simulink model "GEMV_Stream_Ex2"  (R2025a)
settings: Solver=VariableStepAuto  StartTime=0.0  StopTime=100  RelTol=1e-3
undefined symbols (not defined in the file): Column, DUT, GEMV_Ex1_Stream, L, major, vsva1596, xcvc1702
libraries: aieUtilities x2, aieDSP x1, vmcUtilities x1
settings Model: Creator=sdegala  LastModifiedBy=sdegala
settings ModelReferenceCC: EnableRefExpFcnMdlSchedulingChecks=on
settings RTWCC: GPUComputeCapability=3.5

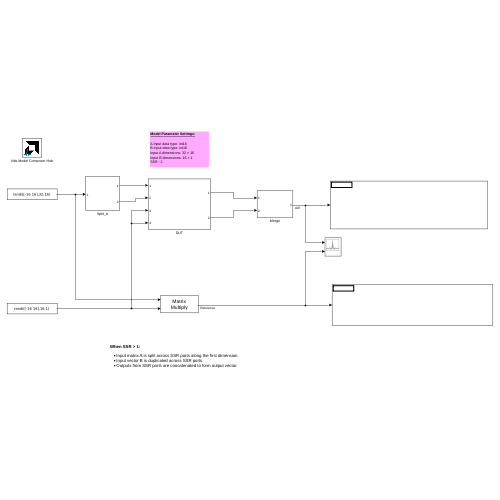
[thumbnail: Simulink's stored preview of the top-level diagram]
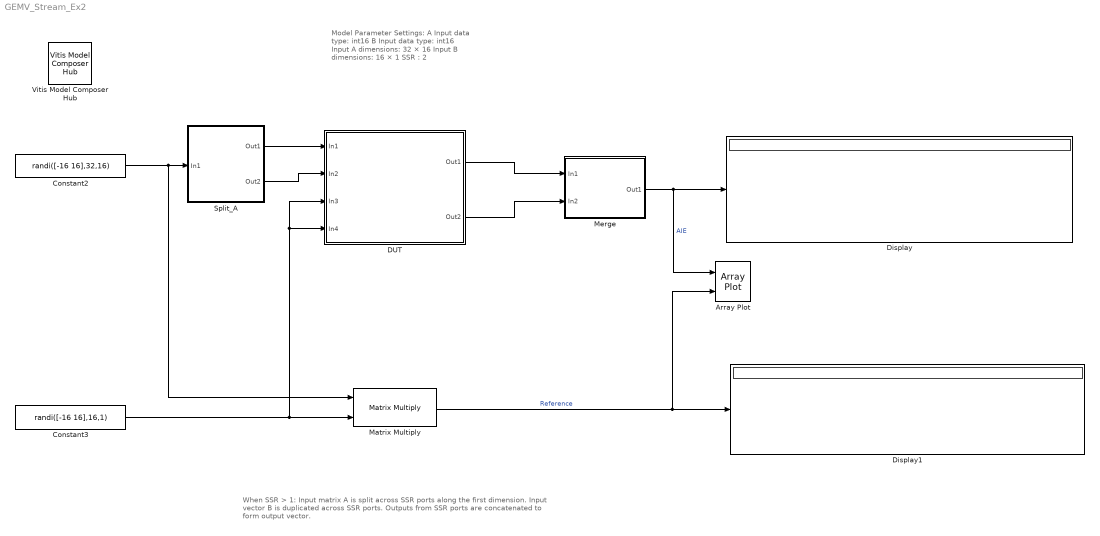
== system GEMV_Stream_Ex2 ==
  note: Model Parameter Settings:
      |
      | A Input data type: int16
      | B Input data type: int16
      | Input A dimensions: 32 × 16
      | Input B dimensions: 16 × 1
      | SSR : 2
  note: When SSR > 1:
      | Input matrix A is split across SSR ports along the first dimension.
      | Input vector B is duplicated across SSR ports.
      | Outputs from SSR ports are concatenated to form output vector.
  Array Plot : ArrayPlot  NumInputPorts=2  WindowPosition=[560.000000,350.000000,800.000000,500.000000,]  Visible=on  ScopeFrameLocation=window  YLimits=[-943.625 1282.625]  ShowLegend=on
  Constant2 : Constant  Value=randi([-16 16],32,16)  OutDataTypeStr=int16  SampleTime=1
  Constant3 : Constant  Value=randi([-16 16],16,1)  OutDataTypeStr=int16  SampleTime=1
  DUT : Subsystem
  Display : Display
  Display1 : Display
  Matrix Multiply : Product  Multiplication=Matrix(*)  OutDataTypeStr=int16
  Merge : Subsystem
  Split_A : Subsystem
  Vitis Model Composer Hub : vmcUtilities/Vitis Model Composer Hub  Tag=genX  CodeGeneration=off  SubsystemName=DUT  BlockHierPath=GEMV_Ex1_Stream/DUT  SubsystemType=AIENode  StartColumn=1  NumberOfColumns=1  TargetDirectory=./code  exportDesign=off  analyzeDesign=on  validateDesignOnHw=off  ExportType=AI Engines  IpVendor=xilinx.com  IpLibrary=hls  IpVersion=1.0  IpHWLanguage=Verilog  AieCompilerOptions={}  AieSimulatorOptions={}  CreateTestbench=on  TestbenchStackSize=10  RunRtlSim=off  RunCSim=off  RunAieSim=off  enableSimulationTimeout=on  enableGraphIterations=on  AieSimTimeout=50000  AieGraphIterations=-1  RunAieSimProfiling=off  LaunchVitisAnalyzer=off  PlotOutput=off  RunX86Sim=off  X86SimTimeout=10  GenHwImage=off  GenLibadfXo=off  GenHwValidationCode=off  PlatformType=Not Specified  HwSystemType=Baremetal  HwValidationTarget=hw  ProjDevice=xcvc1702-vsva1596-2LP-e-L  ProjDevicePart=xcvc1702-vsva1596-2LP-e-L  AIEType=AIE  SamplePeriod=-1  ClockFrequency=200  DataPathParallelism=1  xilinxfamily=versalaicore  part=xcvc1702  speed=-2LP-e-L  package=vsva1596  directory=./netlist  testbench=off  incr_netlist=off  synthesis_tool=Vivado  clock_wrapper=Clock Enables  dbl_ovrd=According to Block Masks  dcm_input_clock_period=10  sysclk_period=10  simulink_period=1  eval_field=0  IPInfoJsonString="{\"DUTSubsystemName\":\"DUT\",\"AIESubsystem\":{\"SubsystemName\":\"DUT\",\"TargetDirectory\":\"./code\",\"AIEArrayConfig\":\"Use entire AIE array\",\"StartColumn\":\"0\",\"NumberOfColumns\":\"1\"},\"SubsystemTag\":\"AIENode\"}"  LogFileName=/proj/xhdhdstaff5/sdegala/Head1/HEAD/2026_1_Work/code/model_composer.log  NThreads=4  IPConfigFile=/tmp/vmctmp-16505700046410390857/GEMV_Ex1_Stream_ipconfig.json
  wires:
  Matrix Multiply/1 -> Array Plot/2, Display1/1  "Reference"
  Constant2/1 -> Matrix Multiply/1, Split_A/1(In1)
  Constant3/1 -> Matrix Multiply/2, DUT/3(In3), DUT/4(In4)
  Split_A/1(Out1) -> DUT/1(In1)
  Split_A/2(Out2) -> DUT/2(In2)
  DUT/1(Out1) -> Merge/1(In1)
  DUT/2(Out2) -> Merge/2(In2)
  Merge/1(Out1) -> Array Plot/1, Display/1  "AIE"

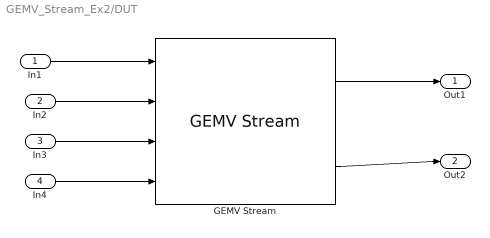
== system GEMV_Stream_Ex2/DUT ==
  In1 : Inport
  In2 : Inport  Port=2
  In3 : Inport  Port=3
  In4 : Inport  Port=4
  GEMV Stream : aieDSP/GEMV Stream  AIE_VARIANT=1  data_type_A=int16  data_type_B=int16  Matrix_reload=on  api=1  Dim_A=32  Dim_B=16  num_frames=1  ssr=2  casc_length=1  dual_ip=off  num_outputs=off  A_Leading_data=Column-major(1)  shift_output=0  rnd_mode=Floor  sat_mode=None  blockJsonConstraints=[]  blockJsonConstraintsInternal=[]  spec=vmc_stream_matrix_vector_mul.json  SerializedMaskParamNames=[]  SerializedMaskParamValues=[]  SerializedMaskParamVisibilities=[]  block_type=GEMV Stream  SerializedMaskParamDataypes=uint|typename|typename|uint|uint|uint|uint|uint|uint|uint|uint|uint|uint|uint|uint|uint  SerializedMaskParamEnumStrArr=0|0|0|0|0|0|0|0|0|0|0|0|Row-major(0),Column-major(1)|0|Floor,Ceiling,Round to positive infinity,Round to negative infinity,Round symmetrical to infinity,Round symmetrical to zero,Round convergent to even,Round convergent to odd|None,Saturate,Symmetric  SerializedMaskParamEnumValArr=0|0|0|0|0|0|0|0|0|0|0|0|0,1|0|0,1,2,3,4,5,6,7|0,1,3  SerializedMaskParamVectorArr=0|0|0|0|0|0|0|0|0|0|0|0|0|0|0|0  SerializedMaskParamKeys=AIE_VARIANT|TT_DATA_A|TT_DATA_B|TP_USE_MATRIX_RELOAD|TP_API|TP_DIM_A|TP_DIM_B|TP_NUM_FRAMES|TP_SSR|TP_CASC_LEN|TP_DUAL_IP|TP_NUM_OUTPUTS|TP_DIM_A_LEADING|TP_SHIFT|TP_RND|TP_SAT
  Out1 : Outport
  Out2 : Outport  Port=2
  wires:
  GEMV Stream/1 -> Out1/1
  In1/1 -> GEMV Stream/1
  In2/1 -> GEMV Stream/2
  In4/1 -> GEMV Stream/4
  In3/1 -> GEMV Stream/3
  GEMV Stream/2 -> Out2/1

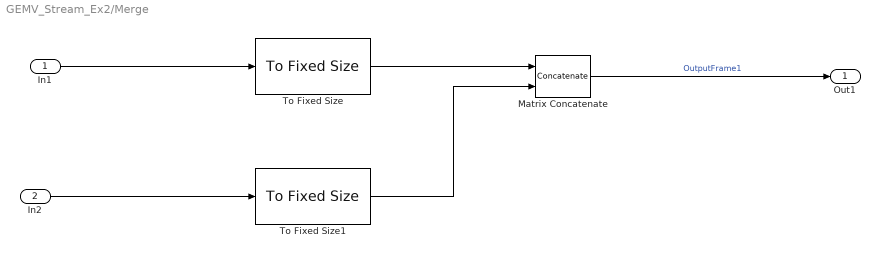
== system GEMV_Stream_Ex2/Merge ==
  In1 : Inport
  In2 : Inport  Port=2
  Matrix Concatenate : Concatenate  ConcatenateDimension=2
  To Fixed Size : aieUtilities/To Fixed Size  Mode=Stop simulation when input variable-size signal is not full  OutputSize=Inherit: Same as input  CopyMethod=Buffer samples to form output  HasStatusOutput=on
  To Fixed Size1 : aieUtilities/To Fixed Size  Mode=Stop simulation when input variable-size signal is not full  OutputSize=Inherit: Same as input  CopyMethod=Buffer samples to form output  HasStatusOutput=on
  Out1 : Outport
  wires:
  To Fixed Size/1 -> Matrix Concatenate/1
  To Fixed Size1/1 -> Matrix Concatenate/2
  Matrix Concatenate/1 -> Out1/1  "OutputFrame1"
  In1/1 -> To Fixed Size/1
  In2/1 -> To Fixed Size1/1

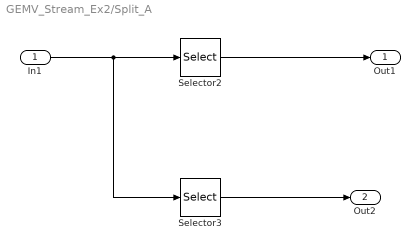
== system GEMV_Stream_Ex2/Split_A ==
  In1 : Inport
  Selector2 : Selector  NumberOfDimensions=2  InputPortWidth=64  IndexOptions=Index vector (dialog),Index vector (dialog)  Indices=1:1:16,1:1:16  OutputSizes=1,1
  Selector3 : Selector  NumberOfDimensions=2  InputPortWidth=64  IndexOptions=Index vector (dialog),Index vector (dialog)  Indices=17:1:32,1:1:16  OutputSizes=1,1
  Out1 : Outport
  Out2 : Outport  Port=2
  wires:
  In1/1 -> Selector3/1, Selector2/1
  Selector2/1 -> Out1/1
  Selector3/1 -> Out2/1
